simulink model "test_PFKV2300"  (R2018b)
settings: Solver=VariableStepAuto  StartTime=0.0  StopTime=10.0  RelTol=1e-3
settings Model: Creator=39926  LastModifiedBy=Administrator

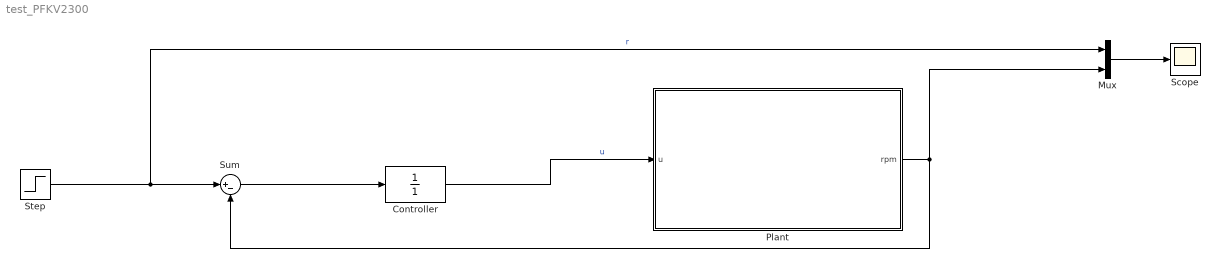
== system test_PFKV2300 ==
  " Controller" : TransferFcn  Denominator=[1]
  Mux : Mux  Inputs=2
  Plant : Subsystem
  Scope : Scope
  Step : Step  After=5000  SampleTime=0
  Sum : Sum  Inputs=|+-
  wires:
  Step/1 -> Mux/1, Sum/1  "r"
  Sum/1 -> " Controller"/1
  " Controller"/1 -> Plant/1(u)  "u"
  Plant/1(rpm) -> Sum/2, Mux/2
  Mux/1 -> Scope/1

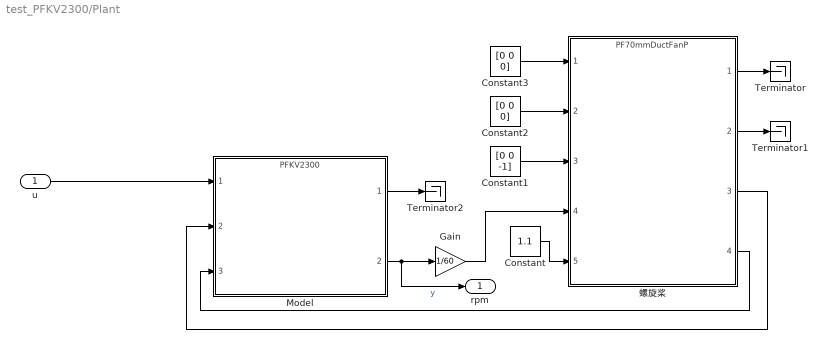
== system test_PFKV2300/Plant ==
  u : Inport
  Constant : Constant  Value=1.1  SampleTime=0.02
  Constant1 : Constant  Value=[0 0 -1]  SampleTime=0.02
  Constant2 : Constant  Value=[0 0 0]  SampleTime=0.02
  Constant3 : Constant  Value=[0 0 0]  SampleTime=0.02
  Gain : Gain  Gain=1/60
  Model : ModelReference  ModelNameDialog=PFKV2300.slx  SimulationMode=Normal  ModelReferenceVersion=1.16
  Terminator : Terminator
  Terminator1 : Terminator
  Terminator2 : Terminator
  螺旋桨 : ModelReference  ModelNameDialog=PF70mmDuctFanP.slx  SimulationMode=Normal  ModelReferenceVersion=1.37
  rpm : Outport
  wires:
  Gain/1 -> 螺旋桨/4
  Model/2 -> rpm/1, Gain/1  "y"
  Constant3/1 -> 螺旋桨/1
  Constant1/1 -> 螺旋桨/3
  Constant2/1 -> 螺旋桨/2
  螺旋桨/4 -> Model/3
  Constant/1 -> 螺旋桨/5
  螺旋桨/3 -> Model/2
  Model/1 -> Terminator2/1
  螺旋桨/2 -> Terminator1/1
  螺旋桨/1 -> Terminator/1
  u/1 -> Model/1
